simulink model "VehCtrlMdel241025_2018b_amkspdlimit"  (R2019b)
settings: Solver=FixedStepDiscrete  StartTime=0.0  StopTime=30  FixedStep=0.0005  RelTol=1e-3  EnableMultiTasking=on
values from neighbouring files (symbols this model uses):
  Ldwf = 0.4    [VxSpdEstiPara.m]
  Ldwr = 0.5    [VxSpdEstiPara.m]
  thr1 = 0.5    [VxSpdEstiPara.m]
  thr2 = 0.5    [VxSpdEstiPara.m]
  thr3 = 0.5    [VxSpdEstiPara.m]
  thr4 = 0.5    [VxSpdEstiPara.m]
  TrqRquRate = 20    [VxSpdEstiPara.m]
undefined symbols (not defined in the file or in its folder): Ax_OffSet, Ay_OffSet, Caf, Car, DiscIntNeverNeededParam, dwf, dwr, h, i1, i2, I_AN06_5V, I_AN07_5V, I_AN08_5V, I_AN09_5V, I_AN10_5V, I_SW01_L, I_SW02_L, I_SW03_L, I_SW05_L, I_SW07_L, Iz, Kc, Ki, Kp, lf, lr, m, O_SW01_LS0A4, O_SW02_LS0A4, O_SW04_LS0A4, O_SW05_LS0A4, O_SW06_LS0A4, O_SW07_LS0A4, O_SW08_LS0A4, O_SW09_LS0A4, O_SW12_HS1A, O_SW13_HS1A, O_SW14_HS1A, O_SW15_HS1A, Offset_Angle, PWM3, Qa, Ra, RearRatio, Rt, thr5, YawRate_OffSet
libraries: simulink x159, ec5744lib x142, canmsglib x18, MyDesignedModel x1
(part 5 of 6)

== system VehCtrlMdel241025_2018b_amkspdlimit/Input/EMRAXMCU_RECIEVE/MCU_pwr/MCU_VCUMeter1 ==
  ID : Inport
  Msg : Inport  Port=2
  Enable : EnablePort
  CAN Unpack : canmsglib/CAN Unpack  CANdbFile=E:\candbc\MCU_No1.dbc  MsgList=(none)  MsgName=MCU2VCU2_ID1  MsgIDType=Extended (29-bit identifier)  MsgIdentifier=218089455  MsgLength=8  SignalInfo={'MCU2VCU2_Current_AC_Feedback_ID1','48','16','LE','unsigned','Standard','0','1.000000e-01','-1600','-1600','1600';'MCU2VCU2_Current_DC_feedback_ID1','32','16','LE','unsigned','Standard','0','1.000000e-01','-1600','-1600','1600';'MCU2VCU2_MCU_Temp_ID1','0','8','LE','unsigned','Standard','0','1','-50','-50','200';'MCU2VCU2_Motor_Temp_ID1','8','8','LE','unsigned','Standard','0','1','-50','-50','200';'MCU2VCU2_Voltage_Feedback_ID1','16','16','LE','unsigned','Standard','0','1.000000e-01','0','0','1000'}  IDPort=off  TimestampPort=off  ErrorPort=off  RemotePort=off  LengthPort=off  StatusPort=off  ApplyMinMax=off
      settings: SourceProductName=Vehicle Network Toolbox  SourceProductBaseCode=VN  DataFormat=CANdb specified signals
  CANUnPackMessage4 : ec5744lib/RapidECU_U3/04CANCommunication/CANUnPackMessage  datalength=8  canmessagetype=Extended(29-bit ID)  sampletime=-1
      settings: SourceProductName=ECUCoder for MPC5744
  MeaModule1 : ec5744lib/RapidECU_U3/07Calibration/MeaModule  signal=AC_current
      settings: SourceProductName=ECUCoder for MPC5744
  MeaModule2 : ec5744lib/RapidECU_U3/07Calibration/MeaModule  signal=DC_current
      settings: SourceProductName=ECUCoder for MPC5744
  MeaModule3 : ec5744lib/RapidECU_U3/07Calibration/MeaModule  signal=MCU_Temp
      settings: SourceProductName=ECUCoder for MPC5744
  MeaModule4 : ec5744lib/RapidECU_U3/07Calibration/MeaModule  signal=motor_Temp
      settings: SourceProductName=ECUCoder for MPC5744
  MeaModule5 : ec5744lib/RapidECU_U3/07Calibration/MeaModule  signal=voltage
      settings: SourceProductName=ECUCoder for MPC5744
  "AC_current " : Outport
  MCU_temp : Outport  Port=2
  current : Outport  Port=3
  motor_temp : Outport  Port=4
  voltage : Outport  Port=5
  wires:
  Msg/1 -> CANUnPackMessage4/2
  ID/1 -> CANUnPackMessage4/1
  CANUnPackMessage4/1 -> CAN Unpack/1
  CAN Unpack/1 -> MeaModule1/1  "AC_current"
  CAN Unpack/5 -> MeaModule5/1  "voltage"
  CAN Unpack/4 -> MeaModule4/1  "moter_temp"
  MeaModule1/1 -> "AC_current "/1
  MeaModule2/1 -> current/1
  CAN Unpack/3 -> MeaModule3/1  "MCU_temp"
  CAN Unpack/2 -> MeaModule2/1  "DC_current"
  MeaModule3/1 -> MCU_temp/1
  MeaModule4/1 -> motor_temp/1
  MeaModule5/1 -> voltage/1

== system VehCtrlMdel241025_2018b_amkspdlimit/Input/EMRAXMCU_RECIEVE/MCU_state/MCU_state ==
  ID : Inport
  Msg : Inport  Port=2
  Enable : EnablePort
  CAN Unpack : canmsglib/CAN Unpack  CANdbFile=E:\candbc\MCU_No1.dbc  MsgList=(none)  MsgName=MCU2VCU1_ID1  MsgIDType=Extended (29-bit identifier)  MsgIdentifier=218089199  MsgLength=8  SignalInfo={'MCU2VCU1_12V_error_ID1','45','1','LE','unsigned','Standard','0','1','0','0','1';'MCU2VCU1_Error_All_ID1','56','2','LE','unsigned','Standard','0','1','0','0','3';'MCU2VCU1_LowVoltage_error_ID1','46','1','LE','unsigned','Standard','0','1','0','0','1';'MCU2VCU1_MCU_Ready_ID1','40','1','LE','unsigned','Standard','0','1','0','0','1';'MCU2VCU1_MCU_Temp_error_ID1','48','1','LE','unsigned','Standard','0','1','0','0','1';'MCU2VCU1_Mode_Feedback_ID1','32','8','LE','unsigned','Standard','0','1','0','0','255';'MCU2VCU1_MotorTemp_error_ID1','49','1','LE','unsigned','Standard','0','1','0','0','1';'MCU2VCU1_OverCurrent_error_ID1','43','1','LE','unsigned','Standard','0','1','0','0','1';'MCU2VCU1_OverPower_error_ID1','47','1','LE','unsigned','Standard','0','1','0','0','1';'MCU2VCU1_OverVoltage_error_ID1','44','1','LE','unsigned','Standard','0','1','0','0','1';'MCU2VCU1_PrechargeState_ID1','41','1','LE','unsigned','Standard','0','1','0','0','1';'MCU2VCU1_Reslove_Error_ID1','42','1','LE','unsigned','Standard','0','1','0','0','1';'MCU2VCU1_Selfcheck_ID1','55','1','LE','unsigned','Standard','0','1','0','0','1';'MCU2VCU1_Speed_Feedback_ID1','0','16','LE','unsigned','Standard','0','5.000000e-01','-10000','-10000','10000';'MCU2VCU1_Torque_Feedback_ID1','16','16','LE','unsigned','Standard','0','1','0','0','1000'}  IDPort=off  TimestampPort=off  ErrorPort=off  RemotePort=off  LengthPort=off  StatusPort=off  ApplyMinMax=off
      settings: SourceProductName=Vehicle Network Toolbox  SourceProductBaseCode=VN  DataFormat=CANdb specified signals
  CANUnPackMessage4 : ec5744lib/RapidECU_U3/04CANCommunication/CANUnPackMessage  datalength=8  canmessagetype=Extended(29-bit ID)  sampletime=-1
      settings: SourceProductName=ECUCoder for MPC5744
  MeaModule : ec5744lib/RapidECU_U3/07Calibration/MeaModule  signal=RPM
      settings: SourceProductName=ECUCoder for MPC5744
  MeaModule1 : ec5744lib/RapidECU_U3/07Calibration/MeaModule  signal=alarm
      settings: SourceProductName=ECUCoder for MPC5744
  MeaModule2 : ec5744lib/RapidECU_U3/07Calibration/MeaModule  signal=L12V_error
      settings: SourceProductName=ECUCoder for MPC5744
  MeaModule3 : ec5744lib/RapidECU_U3/07Calibration/MeaModule  signal=controller_ready
      settings: SourceProductName=ECUCoder for MPC5744
  MeaModule5 : ec5744lib/RapidECU_U3/07Calibration/MeaModule  signal=selfcheck
      settings: SourceProductName=ECUCoder for MPC5744
  MeaModule6 : ec5744lib/RapidECU_U3/07Calibration/MeaModule  signal=trq
      settings: SourceProductName=ECUCoder for MPC5744
  12V_error : Outport
  alarm : Outport  Port=2
  undervol : Outport  Port=3
  controller_ready : Outport  Port=4
  MCU_temp_warn : Outport  Port=5
  mode_cmd8 : Outport  Port=6
  motor_temp_warn : Outport  Port=7
  overcur : Outport  Port=8
  pow_lim_warn : Outport  Port=9
  overvol : Outport  Port=10
  precharge : Outport  Port=11
  rotation_warn : Outport  Port=12
  selfcech : Outport  Port=13
  RPM : Outport  Port=14
  torque : Outport  Port=15
  wires:
  Msg/1 -> CANUnPackMessage4/2
  ID/1 -> CANUnPackMessage4/1
  CANUnPackMessage4/1 -> CAN Unpack/1
  MeaModule/1 -> RPM/1  "RPM"
  MeaModule1/1 -> alarm/1
  MeaModule2/1 -> 12V_error/1
  MeaModule3/1 -> controller_ready/1
  MeaModule5/1 -> selfcech/1
  MeaModule6/1 -> torque/1  "Trq"
  CAN Unpack/14 -> MeaModule/1  "RPM"
  CAN Unpack/15 -> MeaModule6/1  "Trq"
  CAN Unpack/13 -> MeaModule5/1
  CAN Unpack/11 -> precharge/1  "Precharge"
  CAN Unpack/10 -> overvol/1  "overvol"
  CAN Unpack/9 -> pow_lim_warn/1  "overpower"
  CAN Unpack/8 -> overcur/1  "overCurrent"
  CAN Unpack/7 -> motor_temp_warn/1  "motorTemp_error"
  CAN Unpack/6 -> mode_cmd8/1  "Mode"
  CAN Unpack/5 -> MCU_temp_warn/1  "MCU_Temp_error"
  CAN Unpack/4 -> MeaModule3/1  "MCU_Ready"
  CAN Unpack/3 -> undervol/1  "low_VOL"
  CAN Unpack/2 -> MeaModule1/1  "Error_ALL"
  CAN Unpack/1 -> MeaModule2/1  "12V_error"
  CAN Unpack/12 -> rotation_warn/1  "Reslove_error"

== system VehCtrlMdel241025_2018b_amkspdlimit/Input/IMU_Recieve/IMU_state/MCU_state ==
  ID : Inport
  Msg : Inport  Port=2
  Enable : EnablePort
  CAN Unpack : canmsglib/CAN Unpack  CANdbFile=d:\Users\YJR\Desktop\IMU.dbc  MsgList=(none)  MsgName=IMU  MsgIDType=Standard (11-bit identifier)  MsgIdentifier=513  MsgLength=8  SignalInfo={'IMU_Ax_Valid','1','1','LE','unsigned','Standard','0','1','0','-Inf','Inf';'IMU_Ax_Value','40','16','LE','unsigned','Standard','0','1.500000e-04','-4.915200e+00','-Inf','Inf';'IMU_Ay_Valid','2','1','LE','unsigned','Standard','0','1','0','-Inf','Inf';'IMU_Ay_Value','24','16','LE','unsigned','Standard','0','1.500000e-04','-4.915200e+00','-Inf','Inf';'IMU_DTC','4','4','LE','unsigned','Standard','0','1','0','-Inf','Inf';'IMU_Yaw_Valid','3','1','LE','unsigned','Standard','0','1','0','-Inf','Inf';'IMU_Yaw_Value','8','16','LE','unsigned','Standard','0','5.710000e-03','-1.872400e+02','-Inf','Inf'}  IDPort=off  TimestampPort=off  ErrorPort=off  RemotePort=off  LengthPort=off  StatusPort=off  ApplyMinMax=off
      settings: SourceProductName=Simulink Real-Time  SourceProductBaseCode=XP  DataFormat=CANdb specified signals
  CANUnPackMessage4 : ec5744lib/RapidECU_U3/04CANCommunication/CANUnPackMessage  datalength=8  canmessagetype=Standard(11-bit ID)  sampletime=-1
      settings: SourceProductName=ECUCoder for MPC5744
  MeaModule2 : ec5744lib/RapidECU_U3/07Calibration/MeaModule  signal=IMU_Ay_Value
      settings: SourceProductName=ECUCoder for MPC5744
  MeaModule3 : ec5744lib/RapidECU_U3/07Calibration/MeaModule  signal=IMU_Yaw_Value
      settings: SourceProductName=ECUCoder for MPC5744
  MeaModule4 : ec5744lib/RapidECU_U3/07Calibration/MeaModule  signal=IMU_Ax_Value
      settings: SourceProductName=ECUCoder for MPC5744
  IMU_Ax_Value : Outport  VectorParamsAs1DForOutWhenUnconnected=off
  IMU_Ay_Value : Outport  Port=2  VectorParamsAs1DForOutWhenUnconnected=off
  IMU_Yaw_Value : Outport  Port=3  VectorParamsAs1DForOutWhenUnconnected=off
  IMU_Ay_Valid : Outport  Port=4  VectorParamsAs1DForOutWhenUnconnected=off
  IMU_DTC : Outport  Port=5  VectorParamsAs1DForOutWhenUnconnected=off
  IMU_Yaw_Valid : Outport  Port=6  VectorParamsAs1DForOutWhenUnconnected=off
  IMU_Ax_Valid : Outport  Port=7  VectorParamsAs1DForOutWhenUnconnected=off
  wires:
  Msg/1 -> CANUnPackMessage4/2
  ID/1 -> CANUnPackMessage4/1
  CANUnPackMessage4/1 -> CAN Unpack/1
  CAN Unpack/2 -> MeaModule2/1
  CAN Unpack/3 -> IMU_Ay_Valid/1
  CAN Unpack/4 -> MeaModule4/1
  CAN Unpack/5 -> IMU_DTC/1
  CAN Unpack/7 -> MeaModule3/1
  CAN Unpack/6 -> IMU_Yaw_Valid/1
  CAN Unpack/1 -> IMU_Ax_Valid/1
  MeaModule2/1 -> IMU_Ax_Value/1
  MeaModule3/1 -> IMU_Yaw_Value/1
  MeaModule4/1 -> IMU_Ay_Value/1

== system VehCtrlMdel241025_2018b_amkspdlimit/Input/StrSnis_Receive/StrWhSnis_state/IMU_state ==
  ID : Inport
  Msg : Inport  Port=2
  Enable : EnablePort
  CAN Unpack : canmsglib/CAN Unpack  Commented=on  CANdbFile=d:\Users\YJR\Desktop\DBC\SWAS_3.dbc  MsgList=(none)  MsgName=PPEI_Steering_Wheel_Angle  MsgIDType=Standard (11-bit identifier)  MsgIdentifier=330  MsgLength=8  SignalInfo={'SAS_CheckSum','36','4','LE','unsigned','Standard','0','1','0','-Inf','Inf';'SAS_MassageCounter','32','4','LE','unsigned','Standard','0','1','0','0','15';'SAS_TrimmingFlag','26','1','LE','unsigned','Standard','0','1','0','0','255';'StrWhAng','8','16','BE','unsigned','Standard','0','1','0','0','65535';'StrWhAngV','16','8','LE','unsigned','Standard','0','1','0','0','1';'StrWhlAngSenCalFlag','25','1','LE','unsigned','Standard','0','1','0','0','3';'StrngWhlAngSnsrFailFlag','24','1','LE','unsigned','Standard','0','1','0','0','1'}  IDPort=off  TimestampPort=off  ErrorPort=off  RemotePort=off  LengthPort=off  StatusPort=off  ApplyMinMax=off
      settings: SourceProductName=Simulink Real-Time  SourceProductBaseCode=XP  DataFormat=CANdb specified signals
  CAN Unpack1 : canmsglib/CAN Unpack  CANdbFile=d:\Users\YJR\Desktop\DBC\SWAS.dbc  MsgList=(none)  MsgName=PPEI_Steering_Wheel_Angle  MsgIDType=Standard (11-bit identifier)  MsgIdentifier=330  MsgLength=8  SignalInfo={'StWhlAngAliveRollCnt','0','8','BE','unsigned','Standard','0','1','0','0','63';'StrWhAng','32','16','BE','unsigned','Standard','0','0.1','-779.3','-779.3','5774.2';'StrWhAngV','16','8','BE','unsigned','Standard','0','1','0','0','255'}  IDPort=off  TimestampPort=off  ErrorPort=off  RemotePort=off  LengthPort=off  StatusPort=off  ApplyMinMax=off
      settings: SourceProductName=Simulink Real-Time  SourceProductBaseCode=XP  DataFormat=CANdb specified signals
  CANUnPackMessage4 : ec5744lib/RapidECU_U3/04CANCommunication/CANUnPackMessage  datalength=8  canmessagetype=Standard(11-bit ID)  sampletime=-1
      settings: SourceProductName=ECUCoder for MPC5744
  MeaModule1 : ec5744lib/RapidECU_U3/07Calibration/MeaModule  signal=StrWhlAngAliveRollCnt
      settings: SourceProductName=ECUCoder for MPC5744
  MeaModule2 : ec5744lib/RapidECU_U3/07Calibration/MeaModule  signal=StrWhlAng
      settings: SourceProductName=ECUCoder for MPC5744
  MeaModule3 : ec5744lib/RapidECU_U3/07Calibration/MeaModule  signal=StrWhlAngV
      settings: SourceProductName=ECUCoder for MPC5744
  StrWhlAng : Outport  VectorParamsAs1DForOutWhenUnconnected=off
  StrWhlAngV : Outport  Port=2  VectorParamsAs1DForOutWhenUnconnected=off
  StrWhlAngAliveRollCnt : Outport  Port=3  VectorParamsAs1DForOutWhenUnconnected=off
  wires:
  Msg/1 -> CANUnPackMessage4/2
  ID/1 -> CANUnPackMessage4/1
  CANUnPackMessage4/1 -> CAN Unpack1/1
  CAN Unpack1/1 -> MeaModule1/1
  CAN Unpack1/2 -> MeaModule2/1
  CAN Unpack1/3 -> MeaModule3/1
  MeaModule1/1 -> StrWhlAngAliveRollCnt/1
  MeaModule2/1 -> StrWhlAng/1
  MeaModule3/1 -> StrWhlAngV/1

== system VehCtrlMdel241025_2018b_amkspdlimit/Input_Processing/Function-Call Subsystem/IMU/Subsystem ==
  note: 定义数据类型
  IMU_Ax_Value : Inport
  IMU_Ay_Value : Inport  Port=2
  IMU_Yaw_Value : Inport  Port=3
  Add{,1..5} (6 alike) : Sum
  Constant : Constant  Value=5000
  Constant1 : Constant  Value=-5000
  Constant10 : Constant  Value=200  SampleTime=-1
  Constant11 : Constant  Value=-200  SampleTime=-1
  Constant12 : Constant  Value=Ax_OffSet
  Constant13 : Constant  Value=Ay_OffSet
  Constant14 : Constant  Value=YawRate_OffSet
  Constant15 : Constant  Value=Offset_Angle
  Constant16 : Constant  Value=Offset_Angle
  Constant2 : Constant  Value=5000
  Constant3 : Constant  Value=5000
  Constant4 : Constant  Value=-5000
  Constant5 : Constant  Value=-5000
  Constant6 : Constant  Value=1.5  SampleTime=-1
  Constant7 : Constant  Value=-1.5  SampleTime=-1
  Constant8 : Constant  Value=1.5  SampleTime=-1
  Constant9 : Constant  Value=-1.5  SampleTime=-1
  Cos : Trigonometry  Operator=cos
  Cos1 : Trigonometry  Operator=cos
  Gain : Gain  Gain=0.7
  Gain1 : Gain  Gain=0.3
  Gain2 : Gain  Gain=0.7
  Gain3 : Gain  Gain=0.3
  Gain4 : Gain  Gain=0.7
  Gain5 : Gain  Gain=0.3
  Product : Product
  Product1 : Product
  Rate Limiter Dynamic : simulink/Discontinuities/Rate Limiter Dynamic
      settings: SourceProductName=Simulink
  Rate Limiter Dynamic1 : simulink/Discontinuities/Rate Limiter Dynamic
      settings: SourceProductName=Simulink
  Rate Limiter Dynamic2 : simulink/Discontinuities/Rate Limiter Dynamic
      settings: SourceProductName=Simulink
  Saturation Dynamic : simulink/Discontinuities/Saturation Dynamic  OutMin=[]  OutMax=[]  OutDataTypeStr=Inherit: Same as second input  OutDataType=fixdt(1, 16)  OutScaling=2^-10  DoSatur=off
  Saturation Dynamic1 : simulink/Discontinuities/Saturation Dynamic  OutMin=[]  OutMax=[]  OutDataTypeStr=Inherit: Same as second input  OutDataType=fixdt(1, 16)  OutScaling=2^-10  DoSatur=off
  Saturation Dynamic2 : simulink/Discontinuities/Saturation Dynamic  OutMin=[]  OutMax=[]  OutDataTypeStr=Inherit: Same as second input  OutDataType=fixdt(1, 16)  OutScaling=2^-10  DoSatur=off
  Saturation2 : Saturate  UpperLimit=180  LowerLimit=-180
  Unit Delay : UnitDelay  SampleTime=-1  HasFrameUpgradeWarning=on
  Unit Delay1 : UnitDelay  SampleTime=-1  HasFrameUpgradeWarning=on
  Unit Delay2 : UnitDelay  SampleTime=-1  HasFrameUpgradeWarning=on
  IMU_Ax_Value_out : Outport  VectorParamsAs1DForOutWhenUnconnected=off
  IMU_Ay_Value_out : Outport  Port=2  VectorParamsAs1DForOutWhenUnconnected=off
  IMU_Yaw_Value_out : Outport  Port=3  VectorParamsAs1DForOutWhenUnconnected=off
  wires:
  IMU_Ay_Value/1 -> Unit Delay1/1, Gain2/1  "Ay"
  Unit Delay/1 -> Gain1/1
  Gain/1 -> Add2/2
  Constant2/1 -> Rate Limiter Dynamic1/1
  Constant/1 -> Rate Limiter Dynamic/1
  Add2/1 -> Rate Limiter Dynamic/2
  Gain2/1 -> Add1/1
  IMU_Yaw_Value/1 -> Gain4/1, Unit Delay2/1  "YawRate"
  Gain1/1 -> Add2/1
  Gain5/1 -> Add3/2
  IMU_Ax_Value/1 -> Gain/1, Unit Delay/1  "Ax"
  Constant11/1 -> Saturation Dynamic2/3
  Add1/1 -> Rate Limiter Dynamic1/2
  Unit Delay1/1 -> Gain3/1
  Constant8/1 -> Saturation Dynamic1/1
  Add3/1 -> Rate Limiter Dynamic2/2
  Constant4/1 -> Rate Limiter Dynamic1/3
  Rate Limiter Dynamic1/1 -> Saturation Dynamic1/2
  Constant1/1 -> Rate Limiter Dynamic/3
  Gain4/1 -> Add3/1
  Constant7/1 -> Saturation Dynamic/3
  Constant3/1 -> Rate Limiter Dynamic2/1
  Product/1 -> IMU_Ax_Value_out/1  "IMU_Ax_Value"
  Constant9/1 -> Saturation Dynamic1/3
  Add5/1 -> IMU_Yaw_Value_out/1  "IMU_Yaw_Value"
  Rate Limiter Dynamic2/1 -> Saturation2/1
  Saturation2/1 -> Saturation Dynamic2/2  "IMU_Yaw_Value"
  Constant10/1 -> Saturation Dynamic2/1
  Constant5/1 -> Rate Limiter Dynamic2/3
  Rate Limiter Dynamic/1 -> Saturation Dynamic/2
  Gain3/1 -> Add1/2
  Product1/1 -> IMU_Ay_Value_out/1  "IMU_Ay_Value"
  Constant6/1 -> Saturation Dynamic/1
  Unit Delay2/1 -> Gain5/1
  Saturation Dynamic/1 -> Add/1  "IMU_Ax_Value"
  Constant12/1 -> Add/2
  Saturation Dynamic1/1 -> Add4/1  "IMU_Ay_Value"
  Constant13/1 -> Add4/2
  Saturation Dynamic2/1 -> Add5/1  "IMU_Yaw_Value"
  Constant14/1 -> Add5/2
  Add/1 -> Product/1
  Cos/1 -> Product/2
  Constant15/1 -> Cos/1
  Constant16/1 -> Cos1/1
  Cos1/1 -> Product1/2
  Add4/1 -> Product1/1

== system VehCtrlMdel241025_2018b_amkspdlimit/Input_Processing/Subsystem/WhlSlpageJudgment/加速度差判断 ==
  note: 输出“1”代表判定有效
  <VxFL_mps> : Inport
  <VxFR_mps> : Inport  Port=2
  <VxRL_mps> : Inport  Port=3
  <VxRR_mps> : Inport  Port=4
  IMU_Ax_mpss : Inport  Port=5
  Abs{,1..3} (4 alike) : Abs
  Add{,1..3} (4 alike) : Sum  Inputs=+-
  Add{4..7} (4 alike) : Sum  Inputs=-+
  Compare To Constant{,1..3} (4 alike) : simulink/Logic and Bit Operations/Compare To Constant  relop=<=  const=thr2  OutDataTypeStr=boolean
  Divide{,1..3} (4 alike) : Product  Inputs=*/
  Filter : Subsystem
  Filter1 : Subsystem
  Filter2 : Subsystem
  Filter3 : Subsystem
  Unit Delay{,1..3} (4 alike) : UnitDelay  SampleTime=-1  HasFrameUpgradeWarning=on
  steptime{,1..3} (4 alike) : Constant  Value=single(0.01)
  y : Outport
  y1 : Outport  Port=2
  y2 : Outport  Port=3
  y3 : Outport  Port=4
  wires:
  Compare To Constant/1 -> y/1
  Compare To Constant2/1 -> y2/1
  Abs2/1 -> Compare To Constant2/1
  Add1/1 -> Abs1/1
  Abs/1 -> Compare To Constant/1
  [IMU_Ax_mpss] -> Add3/2
  [IMU_Ax_mpss] -> Add2/2
  [IMU_Ax_mpss] -> Add/2
  Abs3/1 -> Compare To Constant3/1
  Compare To Constant3/1 -> y3/1
  Compare To Constant1/1 -> y1/1
  [IMU_Ax_mpss] -> Add1/2
  Add/1 -> Abs/1
  Add3/1 -> Abs3/1
  Abs1/1 -> Compare To Constant1/1
  Add2/1 -> Abs2/1
  <VxFL_mps>/1 -> Add4/2, Unit Delay/1
  Unit Delay/1 -> Add4/1
  Add4/1 -> Divide/1
  steptime/1 -> Divide/2
  Divide/1 -> Filter/1(In)
  IMU_Ax_mpss/1 -> [IMU_Ax_mpss]
  steptime1/1 -> Divide1/2
  Add5/1 -> Divide1/1
  Unit Delay1/1 -> Add5/1
  <VxFR_mps>/1 -> Unit Delay1/1, Add5/2
  Divide1/1 -> Filter1/1(In)
  steptime2/1 -> Divide2/2
  Add6/1 -> Divide2/1
  Unit Delay2/1 -> Add6/1
  <VxRL_mps>/1 -> Unit Delay2/1, Add6/2
  Divide2/1 -> Filter2/1(In)
  steptime3/1 -> Divide3/2
  Add7/1 -> Divide3/1
  Unit Delay3/1 -> Add7/1
  <VxRR_mps>/1 -> Unit Delay3/1, Add7/2
  Divide3/1 -> Filter3/1(In)
  Filter/1(Out) -> Add/1
  Filter1/1(Out) -> Add1/1
  Filter2/1(Out) -> Add2/1
  Filter3/1(Out) -> Add3/1

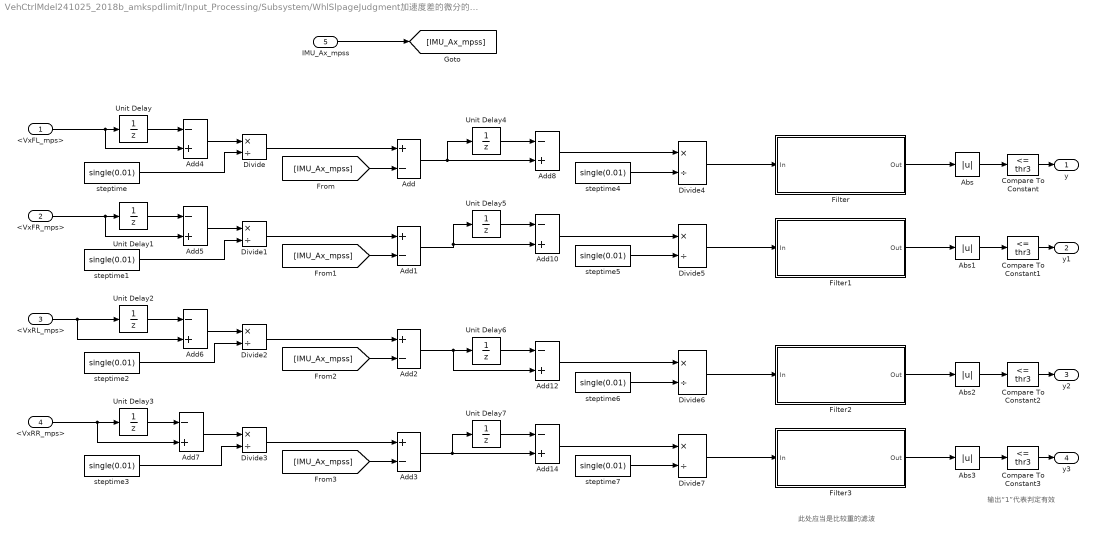
== system VehCtrlMdel241025_2018b_amkspdlimit/Input_Processing/Subsystem/WhlSlpageJudgment/加速度差的微分的判断 ==
  note: 此处应当是比较重的滤波
  note: 输出“1”代表判定有效
  <VxFL_mps> : Inport
  <VxFR_mps> : Inport  Port=2
  <VxRL_mps> : Inport  Port=3
  <VxRR_mps> : Inport  Port=4
  IMU_Ax_mpss : Inport  Port=5
  Abs{,1..3} (4 alike) : Abs
  Add{,1..3} (4 alike) : Sum  Inputs=+-
  Add{4..8,10,12,14} (8 alike) : Sum  Inputs=-+
  Compare To Constant{,1..3} (4 alike) : simulink/Logic and Bit Operations/Compare To Constant  relop=<=  const=thr3  OutDataTypeStr=boolean
  Divide{,1..7} (8 alike) : Product  Inputs=*/
  Filter : Subsystem
  Filter1 : Subsystem
  Filter2 : Subsystem
  Filter3 : Subsystem
  Unit Delay{,1..7} (8 alike) : UnitDelay  SampleTime=-1  HasFrameUpgradeWarning=on
  steptime{,1..7} (8 alike) : Constant  Value=single(0.01)
  y : Outport
  y1 : Outport  Port=2
  y2 : Outport  Port=3
  y3 : Outport  Port=4
  wires:
  Divide3/1 -> Add3/1
  <VxRR_mps>/1 -> Add7/2, Unit Delay3/1
  Unit Delay3/1 -> Add7/1
  Add7/1 -> Divide3/1
  steptime3/1 -> Divide3/2
  Divide2/1 -> Add2/1
  <VxRL_mps>/1 -> Add6/2, Unit Delay2/1
  Unit Delay2/1 -> Add6/1
  Add6/1 -> Divide2/1
  steptime2/1 -> Divide2/2
  Divide1/1 -> Add1/1
  <VxFR_mps>/1 -> Add5/2, Unit Delay1/1
  Unit Delay1/1 -> Add5/1
  Add5/1 -> Divide1/1
  steptime1/1 -> Divide1/2
  IMU_Ax_mpss/1 -> [IMU_Ax_mpss]
  Divide/1 -> Add/1
  steptime/1 -> Divide/2
  Add4/1 -> Divide/1
  Unit Delay/1 -> Add4/1
  <VxFL_mps>/1 -> Unit Delay/1, Add4/2
  Abs1/1 -> Compare To Constant1/1
  [IMU_Ax_mpss] -> Add1/2
  Compare To Constant1/1 -> y1/1
  Compare To Constant3/1 -> y3/1
  Abs3/1 -> Compare To Constant3/1
  [IMU_Ax_mpss] -> Add/2
  [IMU_Ax_mpss] -> Add2/2
  [IMU_Ax_mpss] -> Add3/2
  Abs/1 -> Compare To Constant/1
  Abs2/1 -> Compare To Constant2/1
  Compare To Constant2/1 -> y2/1
  Compare To Constant/1 -> y/1
  Add/1 -> Add8/2, Unit Delay4/1
  Unit Delay4/1 -> Add8/1
  Add8/1 -> Divide4/1
  steptime4/1 -> Divide4/2
  Divide4/1 -> Filter/1(In)
  steptime5/1 -> Divide5/2
  Add10/1 -> Divide5/1
  Unit Delay5/1 -> Add10/1
  Add1/1 -> Unit Delay5/1, Add10/2
  Divide5/1 -> Filter1/1(In)
  Divide6/1 -> Filter2/1(In)
  Add2/1 -> Add12/2, Unit Delay6/1
  Add12/1 -> Divide6/1
  steptime6/1 -> Divide6/2
  Unit Delay6/1 -> Add12/1
  steptime7/1 -> Divide7/2
  Add14/1 -> Divide7/1
  Add3/1 -> Unit Delay7/1, Add14/2
  Unit Delay7/1 -> Add14/1
  Divide7/1 -> Filter3/1(In)
  Filter/1(Out) -> Abs/1
  Filter1/1(Out) -> Abs1/1
  Filter2/1(Out) -> Abs2/1
  Filter3/1(Out) -> Abs3/1

== system VehCtrlMdel241025_2018b_amkspdlimit/Input_Processing/Subsystem/WhlSlpageJudgment/速差判断 ==
  note: 输出“1”代表判定有效
  <VxFL_mps> : Inport
  <VxFR_mps> : Inport  Port=2
  <VxRL_mps> : Inport  Port=3
  <VxRR_mps> : Inport  Port=4
  VehSpd_mps : Inport  Port=5
  In6 : Inport  Port=6
  AND{,1..3} (4 alike) : Logic  AllPortsSameDT=off  OutDataTypeStr=boolean
  Abs{,1..3} (4 alike) : Abs
  Add{,1..3} (4 alike) : Sum  Inputs=+-
  Bus Selector1 : BusSelector  OutputSignals=WhlSpdii_mps.WhlSpdRL_Valid,WhlSpdii_mps.WhlSpdRR_Valid,WhlSpdii_mps.WhlSpdFR_Valid,WhlSpdii_mps.WhlSpdFL_Valid
  Compare To Constant{,1..3} (4 alike) : simulink/Logic and Bit Operations/Compare To Constant  relop=<=  const=thr1  OutDataTypeStr=boolean
  y : Outport
  y1 : Outport  Port=2
  y2 : Outport  Port=3
  y3 : Outport  Port=4
  wires:
  Add2/1 -> Abs2/1
  Abs1/1 -> Compare To Constant1/1
  <VxRR_mps>/1 -> Add3/1
  Add3/1 -> Abs3/1
  Add/1 -> Abs/1
  [VehSpd_mps] -> Add1/2
  <VxRL_mps>/1 -> Add2/1
  <VxFR_mps>/1 -> Add1/1
  Compare To Constant1/1 -> AND2/1
  Compare To Constant3/1 -> AND1/1
  Abs3/1 -> Compare To Constant3/1
  [VehSpd_mps] -> Add/2
  [VehSpd_mps] -> Add2/2
  [VehSpd_mps] -> Add3/2
  Abs/1 -> Compare To Constant/1
  Add1/1 -> Abs1/1
  Abs2/1 -> Compare To Constant2/1
  <VxFL_mps>/1 -> Add/1
  Compare To Constant2/1 -> AND/1
  Compare To Constant/1 -> AND3/1
  VehSpd_mps/1 -> [VehSpd_mps]
  In6/1 -> Bus Selector1/1
  Bus Selector1/1 -> AND/2  "<WhlSpdRL_Valid>"
  Bus Selector1/2 -> AND1/2  "<WhlSpdRR_Valid>"
  Bus Selector1/3 -> AND2/2  "<WhlSpdFR_Valid>"
  Bus Selector1/4 -> AND3/2  "<WhlSpdFL_Valid>"
  AND3/1 -> y/1
  AND2/1 -> y1/1
  AND1/1 -> y3/1
  AND/1 -> y2/1

== system VehCtrlMdel241025_2018b_amkspdlimit/Input_Processing/Subsystem/WhlSpdSelect/Filter ==
  In : Inport
  Add : Sum
  Constant : Constant  Value=single(0)
  Constant1 : Constant  Value=single(100)
  Constant2 : Constant  Value=single(15)
  Constant3 : Constant  Value=single(-15)
  Gain : Gain  Gain=0
  Gain1 : Gain
  Rate Limiter Dynamic : simulink/Discontinuities/Rate Limiter Dynamic
      settings: SourceProductName=Simulink
  Saturation Dynamic : simulink/Discontinuities/Saturation Dynamic  OutMin=[]  OutMax=[]  OutDataTypeStr=Inherit: Same as second input  OutDataType=fixdt(1, 16)  OutScaling=2^-10  DoSatur=off
  Unit Delay : UnitDelay  SampleTime=-1  HasFrameUpgradeWarning=on
  VehVxEst_mps : Outport
  wires:
  In/1 -> Saturation Dynamic/2
  Saturation Dynamic/1 -> Rate Limiter Dynamic/2
  Constant1/1 -> Saturation Dynamic/1
  Constant/1 -> Saturation Dynamic/3
  Unit Delay/1 -> Gain/1
  Gain/1 -> Add/1
  Gain1/1 -> Add/2
  Rate Limiter Dynamic/1 -> Gain1/1, Unit Delay/1
  Add/1 -> VehVxEst_mps/1
  Constant2/1 -> Rate Limiter Dynamic/1
  Constant3/1 -> Rate Limiter Dynamic/3

== system VehCtrlMdel241025_2018b_amkspdlimit/Input_Processing/Subsystem/WhlSpdSelect/Subsystem ==
  <VxFL_mps> : Inport
  <VxFR_mps> : Inport  Port=2
  <VxRL_mps> : Inport  Port=3
  <VxRR_mps> : Inport  Port=4
  Add3 : Sum  Inputs=++++
  Add4 : Sum  Inputs=+--
  Gain1 : Gain  Gain=1/2
  Min3 : MinMax  Function=max  Inputs=4
  Min4 : MinMax  Inputs=4
  Subsystem : Subsystem  Commented=on
  MiddleWhlSpd_mps : Outport
  wires:
  Add4/1 -> Gain1/1
  Add3/1 -> Add4/1
  Min3/1 -> Add4/3
  <VxRR_mps>/1 -> Min3/4, Add3/1, Min4/4
  <VxRL_mps>/1 -> Min3/3, Min4/3, Add3/2
  <VxFR_mps>/1 -> Min4/2, Min3/2, Add3/3
  Min4/1 -> Add4/2
  <VxFL_mps>/1 -> Add3/4, Min4/1, Min3/1
  Gain1/1 -> MiddleWhlSpd_mps/1  "MaxWhlSpd_mps"

== system VehCtrlMdel241025_2018b_amkspdlimit/Input/AMKMCU_Receive/FLAMKMCU/AMKMCU_state/MCU_state ==
  ID : Inport
  Msg : Inport  Port=2
  Enable : EnablePort
  Bus Creator : BusCreator  Inputs=12
  CAN Unpack : canmsglib/CAN Unpack  CANdbFile=d:\Users\YJR\Desktop\低压组\amk电机\DRe20_dbc_v1.16\DRe20_dbc_v1.16_CAN2.dbc  MsgList=(none)  MsgName=MCFL_ActualValue1  MsgIDType=Standard (11-bit identifier)  MsgIdentifier=640  MsgLength=8  SignalInfo={'MCFL_ActualTorque','32','16','LE','signed','Standard','0','0.0098','0','-Inf','Inf';'MCFL_ActualVelocity','48','16','LE','signed','Standard','0','1','0','-Inf','Inf';'MCFL_DCVoltage','16','16','LE','unsigned','Standard','0','1','0','-Inf','Inf';'MCFL_bDCOn','12','1','LE','unsigned','Standard','0','1','0','0','1';'MCFL_bDerating','15','1','LE','unsigned','Standard','0','1','0','0','1';'MCFL_bError','9','1','LE','unsigned','Standard','0','1','0','0','1';'MCFL_bInverterOn','14','1','LE','unsigned','Standard','0','1','0','0','1';'MCFL_bQuitDCOn','11','1','LE','unsigned','Standard','0','1','0','0','1';'MCFL_bQuitInverterOn','13','1','LE','unsigned','Standard','0','1','0','0','1';'MCFL_bReserve','0','8','LE','unsigned','Standard','0','1','0','0','255';'MCFL_bSystemReady','8','1','LE','unsigned','Standard','0','1','0','0','1';'MCFL_bWarn','10','1','LE','unsigned','Standard','0','1','0','0','1'}  IDPort=off  TimestampPort=off  ErrorPort=off  RemotePort=off  LengthPort=off  StatusPort=off  ApplyMinMax=off
      settings: SourceProductName=Simulink Real-Time  SourceProductBaseCode=XP  DataFormat=CANdb specified signals
  CANUnPackMessage4 : ec5744lib/RapidECU_U3/04CANCommunication/CANUnPackMessage  datalength=8  canmessagetype=Standard(11-bit ID)  sampletime=-1
      settings: SourceProductName=ECUCoder for MPC5744
  MeaModule1 : ec5744lib/RapidECU_U3/07Calibration/MeaModule  signal=MCFL_ActualVelocity
      settings: SourceProductName=ECUCoder for MPC5744
  MeaModule2 : ec5744lib/RapidECU_U3/07Calibration/MeaModule  signal=MCFL_DCVoltage
      settings: SourceProductName=ECUCoder for MPC5744
  MeaModule3 : ec5744lib/RapidECU_U3/07Calibration/MeaModule  signal=MCFL_bDCOn
      settings: SourceProductName=ECUCoder for MPC5744
  MeaModule4 : ec5744lib/RapidECU_U3/07Calibration/MeaModule  signal=MCFL_bError
      settings: SourceProductName=ECUCoder for MPC5744
  MeaModule5 : ec5744lib/RapidECU_U3/07Calibration/MeaModule  signal=MCFL_bInverterOn
      settings: SourceProductName=ECUCoder for MPC5744
  MeaModule6 : ec5744lib/RapidECU_U3/07Calibration/MeaModule  signal=MCFL_bQuitDCOn
      settings: SourceProductName=ECUCoder for MPC5744
  MeaModule7 : ec5744lib/RapidECU_U3/07Calibration/MeaModule  signal=MCFL_bQuitInverterOn
      settings: SourceProductName=ECUCoder for MPC5744
  MeaModule8 : ec5744lib/RapidECU_U3/07Calibration/MeaModule  signal=MCFL_bSystemReady
      settings: SourceProductName=ECUCoder for MPC5744
  MeaModule9 : ec5744lib/RapidECU_U3/07Calibration/MeaModule  signal=MCFL_ActualTorque
      settings: SourceProductName=ECUCoder for MPC5744
  FLAMKMCUtoVCU1 : Outport  VectorParamsAs1DForOutWhenUnconnected=off
  wires:
  Msg/1 -> CANUnPackMessage4/2
  ID/1 -> CANUnPackMessage4/1
  CANUnPackMessage4/1 -> CAN Unpack/1
  CAN Unpack/1 -> MeaModule9/1  "MCFL_ActualTorque"
  CAN Unpack/2 -> MeaModule1/1  "MCFL_ActualVelocity"
  CAN Unpack/3 -> MeaModule2/1  "MCFL_DCVoltage"
  CAN Unpack/4 -> MeaModule3/1  "MCFL_bDCOn"
  CAN Unpack/5 -> Bus Creator/5  "MCFL_bDerating"
  CAN Unpack/6 -> MeaModule4/1  "MCFL_bError"
  CAN Unpack/7 -> MeaModule5/1  "MCFL_bInverterOn"
  CAN Unpack/8 -> MeaModule6/1  "MCFL_bQuitDCOn"
  CAN Unpack/9 -> MeaModule7/1  "MCFL_bQuitInverterOn"
  CAN Unpack/10 -> Bus Creator/10  "MCFL_bReserve"
  CAN Unpack/11 -> MeaModule8/1  "MCFL_bSystemReady"
  CAN Unpack/12 -> Bus Creator/12  "MCFL_bWarn"
  Bus Creator/1 -> FLAMKMCUtoVCU1/1  "FLAMKMCUtoVCU1"
  MeaModule1/1 -> Bus Creator/2
  MeaModule2/1 -> Bus Creator/3
  MeaModule3/1 -> Bus Creator/4
  MeaModule4/1 -> Bus Creator/6
  MeaModule5/1 -> Bus Creator/7
  MeaModule6/1 -> Bus Creator/8
  MeaModule7/1 -> Bus Creator/9
  MeaModule8/1 -> Bus Creator/11
  MeaModule9/1 -> Bus Creator/1  "MCFL_ActualTorque"

== system VehCtrlMdel241025_2018b_amkspdlimit/Input/AMKMCU_Receive/FLAMKMCU/AMKMCU_state1/MCU_state ==
  ID : Inport
  Msg : Inport  Port=2
  Enable : EnablePort
  CAN Unpack : canmsglib/CAN Unpack  CANdbFile=d:\Users\YJR\Desktop\低压组\amk电机\DRe20_dbc_v1.16\DRe20_dbc_v1.16_CAN2.dbc  MsgList=(none)  MsgName=MCFL_ActualValue2  MsgIDType=Standard (11-bit identifier)  MsgIdentifier=642  MsgLength=8  SignalInfo={'MCFL_DiagnosticNum','0','32','LE','unsigned','Standard','0','1','0','-Inf','Inf';'MCFL_ErrorInfo','32','32','LE','unsigned','Standard','0','1','0','-Inf','Inf'}  IDPort=off  TimestampPort=off  ErrorPort=off  RemotePort=off  LengthPort=off  StatusPort=off  ApplyMinMax=off
      settings: SourceProductName=Simulink Real-Time  SourceProductBaseCode=XP  DataFormat=CANdb specified signals
  CANUnPackMessage4 : ec5744lib/RapidECU_U3/04CANCommunication/CANUnPackMessage  datalength=8  canmessagetype=Standard(11-bit ID)  sampletime=-1
      settings: SourceProductName=ECUCoder for MPC5744
  MeaModule1 : ec5744lib/RapidECU_U3/07Calibration/MeaModule  signal=MCFL_ErrorInfo
      settings: SourceProductName=ECUCoder for MPC5744
  MCFL_DiagnosticNum : Outport  VectorParamsAs1DForOutWhenUnconnected=off
  MCFL_ErrorInfo : Outport  Port=2  VectorParamsAs1DForOutWhenUnconnected=off
  wires:
  CANUnPackMessage4/1 -> CAN Unpack/1
  ID/1 -> CANUnPackMessage4/1
  Msg/1 -> CANUnPackMessage4/2
  CAN Unpack/1 -> MCFL_DiagnosticNum/1  "MCFL_DiagnosticNum"
  CAN Unpack/2 -> MeaModule1/1  "MCFL_ErrorInfo"
  MeaModule1/1 -> MCFL_ErrorInfo/1

== system VehCtrlMdel241025_2018b_amkspdlimit/Input/AMKMCU_Receive/FLAMKMCU/AMKMCU_state2/MCU_state ==
  ID : Inport
  Msg : Inport  Port=2
  Enable : EnablePort
  CAN Unpack : canmsglib/CAN Unpack  CANdbFile=d:\Users\YJR\Desktop\低压组\amk电机\DRe20_dbc_v1.16\DRe20_dbc_v1.16_CAN2.dbc  MsgList=(none)  MsgName=MCFL_ActualValue3  MsgIDType=Standard (11-bit identifier)  MsgIdentifier=644  MsgLength=6  SignalInfo={'MCFL_TempIGBT','32','16','LE','unsigned','Standard','0','0.1','0','-Inf','Inf';'MCFL_TempInverter','16','16','LE','unsigned','Standard','0','0.1','0','-Inf','Inf';'MCFL_TempMotor','0','16','LE','unsigned','Standard','0','0.1','0','-Inf','Inf'}  IDPort=off  TimestampPort=off  ErrorPort=off  RemotePort=off  LengthPort=off  StatusPort=off  ApplyMinMax=off
      settings: SourceProductName=Simulink Real-Time  SourceProductBaseCode=XP  DataFormat=CANdb specified signals
  CANUnPackMessage4 : ec5744lib/RapidECU_U3/04CANCommunication/CANUnPackMessage  datalength=6  canmessagetype=Standard(11-bit ID)  sampletime=-1
      settings: SourceProductName=ECUCoder for MPC5744
  MeaModule1 : ec5744lib/RapidECU_U3/07Calibration/MeaModule  signal=MCFL_TempIGBT
      settings: SourceProductName=ECUCoder for MPC5744
  MeaModule2 : ec5744lib/RapidECU_U3/07Calibration/MeaModule  signal=MCFL_TempInverter
      settings: SourceProductName=ECUCoder for MPC5744
  MeaModule3 : ec5744lib/RapidECU_U3/07Calibration/MeaModule  signal=MCFL_TempMotor
      settings: SourceProductName=ECUCoder for MPC5744
  MCFL_TempIGBT : Outport  VectorParamsAs1DForOutWhenUnconnected=off
  MCFL_TempInverter : Outport  Port=2  VectorParamsAs1DForOutWhenUnconnected=off
  MCFL_TempMotor : Outport  Port=3  VectorParamsAs1DForOutWhenUnconnected=off
  wires:
  Msg/1 -> CANUnPackMessage4/2
  ID/1 -> CANUnPackMessage4/1
  CANUnPackMessage4/1 -> CAN Unpack/1
  CAN Unpack/1 -> MeaModule1/1  "MCFL_TempIGBT"
  CAN Unpack/2 -> MeaModule2/1  "MCFL_TempInverter"
  CAN Unpack/3 -> MeaModule3/1  "MCFL_TempMotor"
  MeaModule1/1 -> MCFL_TempIGBT/1
  MeaModule2/1 -> MCFL_TempInverter/1
  MeaModule3/1 -> MCFL_TempMotor/1

== system VehCtrlMdel241025_2018b_amkspdlimit/Input/AMKMCU_Receive/FRAMKMCU/AMKMCU_state/MCU_state ==
  ID : Inport
  Msg : Inport  Port=2
  Enable : EnablePort
  CAN Unpack : canmsglib/CAN Unpack  CANdbFile=d:\Users\YJR\Desktop\低压组\amk电机\DRe20_dbc_v1.16\DRe20_dbc_v1.16_CAN2.dbc  MsgList=(none)  MsgName=MCFR_ActualValue1  MsgIDType=Standard (11-bit identifier)  MsgIdentifier=641  MsgLength=8  SignalInfo={'MCFR_ActualTorque','32','16','LE','signed','Standard','0','0.0098','0','-Inf','Inf';'MCFR_ActualVelocity','48','16','LE','signed','Standard','0','1','0','-Inf','Inf';'MCFR_DCVoltage','16','16','LE','unsigned','Standard','0','1','0','-Inf','Inf';'MCFR_bDCOn','12','1','LE','unsigned','Standard','0','1','0','0','1';'MCFR_bDerating','15','1','LE','unsigned','Standard','0','1','0','0','1';'MCFR_bError','9','1','LE','unsigned','Standard','0','1','0','0','1';'MCFR_bInverterOn','14','1','LE','unsigned','Standard','0','1','0','0','1';'MCFR_bQuitDCOn','11','1','LE','unsigned','Standard','0','1','0','0','1';'MCFR_bQuitInverterOn','13','1','LE','unsigned','Standard','0','1','0','0','1';'MCFR_bReserve','0','8','LE','unsigned','Standard','0','1','0','0','255';'MCFR_bSystemReady','8','1','LE','unsigned','Standard','0','1','0','0','1';'MCFR_bWarn','10','1','LE','unsigned','Standard','0','1','0','0','1'}  IDPort=off  TimestampPort=off  ErrorPort=off  RemotePort=off  LengthPort=off  StatusPort=off  ApplyMinMax=off
      settings: SourceProductName=Simulink Real-Time  SourceProductBaseCode=XP  DataFormat=CANdb specified signals
  CANUnPackMessage4 : ec5744lib/RapidECU_U3/04CANCommunication/CANUnPackMessage  datalength=8  canmessagetype=Standard(11-bit ID)  sampletime=-1
      settings: SourceProductName=ECUCoder for MPC5744
  MeaModule1 : ec5744lib/RapidECU_U3/07Calibration/MeaModule  signal=MCFR_ActualVelocity
      settings: SourceProductName=ECUCoder for MPC5744
  MeaModule2 : ec5744lib/RapidECU_U3/07Calibration/MeaModule  signal=MCFR_DCVoltage
      settings: SourceProductName=ECUCoder for MPC5744
  MeaModule3 : ec5744lib/RapidECU_U3/07Calibration/MeaModule  signal=MCFR_bDCOn
      settings: SourceProductName=ECUCoder for MPC5744
  MeaModule4 : ec5744lib/RapidECU_U3/07Calibration/MeaModule  signal=MCFR_bError
      settings: SourceProductName=ECUCoder for MPC5744
  MeaModule5 : ec5744lib/RapidECU_U3/07Calibration/MeaModule  signal=MCFR_bInverterOn
      settings: SourceProductName=ECUCoder for MPC5744
  MeaModule6 : ec5744lib/RapidECU_U3/07Calibration/MeaModule  signal=MCFR_bQuitInverterOn
      settings: SourceProductName=ECUCoder for MPC5744
  MeaModule7 : ec5744lib/RapidECU_U3/07Calibration/MeaModule  signal=MCFR_bSystemReady
      settings: SourceProductName=ECUCoder for MPC5744
  MeaModule8 : ec5744lib/RapidECU_U3/07Calibration/MeaModule  signal=MCFR_ActualTorque
      settings: SourceProductName=ECUCoder for MPC5744
  MCFR_ActualTorque : Outport  VectorParamsAs1DForOutWhenUnconnected=off
  MCFR_ActualVelocity : Outport  Port=2  VectorParamsAs1DForOutWhenUnconnected=off
  MCFR_DCVoltage : Outport  Port=3  VectorParamsAs1DForOutWhenUnconnected=off
  MCFR_bDCOn : Outport  Port=4  VectorParamsAs1DForOutWhenUnconnected=off
  MCFR_bDerating : Outport  Port=5  VectorParamsAs1DForOutWhenUnconnected=off
  MCFR_bError : Outport  Port=6  VectorParamsAs1DForOutWhenUnconnected=off
  MCFR_bInverterOn : Outport  Port=7  VectorParamsAs1DForOutWhenUnconnected=off
  MCFR_bQuitDCOn : Outport  Port=8  VectorParamsAs1DForOutWhenUnconnected=off
  MCFR_bQuitInverterOn : Outport  Port=9  VectorParamsAs1DForOutWhenUnconnected=off
  MCFR_bReserve : Outport  Port=10  VectorParamsAs1DForOutWhenUnconnected=off
  MCFR_bSystemReady : Outport  Port=11  VectorParamsAs1DForOutWhenUnconnected=off
  MCFR_bWarn : Outport  Port=12  VectorParamsAs1DForOutWhenUnconnected=off
  wires:
  CANUnPackMessage4/1 -> CAN Unpack/1
  ID/1 -> CANUnPackMessage4/1
  Msg/1 -> CANUnPackMessage4/2
  CAN Unpack/1 -> MeaModule8/1  "MCFR_ActualTorque"
  CAN Unpack/2 -> MeaModule1/1  "MCFR_ActualVelocity"
  CAN Unpack/4 -> MeaModule3/1  "MCFR_bDCOn"
  CAN Unpack/3 -> MeaModule2/1  "MCFR_DCVoltage"
  CAN Unpack/7 -> MeaModule5/1  "MCFR_bInverterOn"
  CAN Unpack/5 -> MCFR_bDerating/1  "MCFR_bDerating"
  CAN Unpack/6 -> MeaModule4/1  "MCFR_bError"
  CAN Unpack/8 -> MCFR_bQuitDCOn/1  "MCFR_bQuitDCOn"
  CAN Unpack/9 -> MeaModule6/1  "MCFR_bQuitInverterOn"
  CAN Unpack/10 -> MCFR_bReserve/1  "MCFR_bReserve"
  CAN Unpack/11 -> MeaModule7/1  "MCFR_bSystemReady"
  CAN Unpack/12 -> MCFR_bWarn/1  "MCFR_bWarn"
  MeaModule1/1 -> MCFR_ActualVelocity/1
  MeaModule2/1 -> MCFR_DCVoltage/1
  MeaModule3/1 -> MCFR_bDCOn/1
  MeaModule4/1 -> MCFR_bError/1
  MeaModule5/1 -> MCFR_bInverterOn/1
  MeaModule6/1 -> MCFR_bQuitInverterOn/1
  MeaModule7/1 -> MCFR_bSystemReady/1
  MeaModule8/1 -> MCFR_ActualTorque/1  "MCFR_ActualTorque"

== system VehCtrlMdel241025_2018b_amkspdlimit/Input/AMKMCU_Receive/FRAMKMCU/AMKMCU_state1/MCU_state ==
  ID : Inport
  Msg : Inport  Port=2
  Enable : EnablePort
  CAN Unpack : canmsglib/CAN Unpack  CANdbFile=d:\Users\YJR\Desktop\低压组\amk电机\DRe20_dbc_v1.16\DRe20_dbc_v1.16_CAN2.dbc  MsgList=(none)  MsgName=MCFR_ActualValue2  MsgIDType=Standard (11-bit identifier)  MsgIdentifier=643  MsgLength=8  SignalInfo={'MCFR_DiagnosticNum','0','32','LE','unsigned','Standard','0','1','0','-Inf','Inf';'MCFR_ErrorInfo','32','32','LE','unsigned','Standard','0','1','0','-Inf','Inf'}  IDPort=off  TimestampPort=off  ErrorPort=off  RemotePort=off  LengthPort=off  StatusPort=off  ApplyMinMax=off
      settings: SourceProductName=Simulink Real-Time  SourceProductBaseCode=XP  DataFormat=CANdb specified signals
  CANUnPackMessage4 : ec5744lib/RapidECU_U3/04CANCommunication/CANUnPackMessage  datalength=8  canmessagetype=Standard(11-bit ID)  sampletime=-1
      settings: SourceProductName=ECUCoder for MPC5744
  MeaModule1 : ec5744lib/RapidECU_U3/07Calibration/MeaModule  signal=MCFR_ErrorInfo
      settings: SourceProductName=ECUCoder for MPC5744
  MCFR_DiagnosticNum : Outport  VectorParamsAs1DForOutWhenUnconnected=off
  MCFR_ErrorInfo : Outport  Port=2  VectorParamsAs1DForOutWhenUnconnected=off
  wires:
  Msg/1 -> CANUnPackMessage4/2
  ID/1 -> CANUnPackMessage4/1
  CANUnPackMessage4/1 -> CAN Unpack/1
  CAN Unpack/1 -> MCFR_DiagnosticNum/1  "MCFR_DiagnosticNum"
  CAN Unpack/2 -> MeaModule1/1  "MCFR_ErrorInfo"
  MeaModule1/1 -> MCFR_ErrorInfo/1

== system VehCtrlMdel241025_2018b_amkspdlimit/Input/AMKMCU_Receive/FRAMKMCU/AMKMCU_state2/MCU_state ==
  ID : Inport
  Msg : Inport  Port=2
  Enable : EnablePort
  CAN Unpack : canmsglib/CAN Unpack  CANdbFile=d:\Users\YJR\Desktop\低压组\amk电机\DRe20_dbc_v1.16\DRe20_dbc_v1.16_CAN2.dbc  MsgList=(none)  MsgName=MCFR_ActualValue3  MsgIDType=Standard (11-bit identifier)  MsgIdentifier=645  MsgLength=6  SignalInfo={'MCFR_TempIGBT','32','16','LE','unsigned','Standard','0','0.1','0','-Inf','Inf';'MCFR_TempInverter','16','16','LE','unsigned','Standard','0','0.1','0','-Inf','Inf';'MCFR_TempMotor','0','16','LE','unsigned','Standard','0','0.1','0','-Inf','Inf'}  IDPort=off  TimestampPort=off  ErrorPort=off  RemotePort=off  LengthPort=off  StatusPort=off  ApplyMinMax=off
      settings: SourceProductName=Simulink Real-Time  SourceProductBaseCode=XP  DataFormat=CANdb specified signals
  CANUnPackMessage4 : ec5744lib/RapidECU_U3/04CANCommunication/CANUnPackMessage  datalength=6  canmessagetype=Standard(11-bit ID)  sampletime=-1
      settings: SourceProductName=ECUCoder for MPC5744
  MeaModule1 : ec5744lib/RapidECU_U3/07Calibration/MeaModule  signal=MCFR_TempIGBT
      settings: SourceProductName=ECUCoder for MPC5744
  MeaModule2 : ec5744lib/RapidECU_U3/07Calibration/MeaModule  signal=MCFR_TempInverter
      settings: SourceProductName=ECUCoder for MPC5744
  MeaModule3 : ec5744lib/RapidECU_U3/07Calibration/MeaModule  signal=MCFR_TempMotor
      settings: SourceProductName=ECUCoder for MPC5744
  MCFR_TempIGBT : Outport  VectorParamsAs1DForOutWhenUnconnected=off
  MCFR_TempInverter : Outport  Port=2  VectorParamsAs1DForOutWhenUnconnected=off
  MCFR_TempMotor : Outport  Port=3  VectorParamsAs1DForOutWhenUnconnected=off
  wires:
  CANUnPackMessage4/1 -> CAN Unpack/1
  ID/1 -> CANUnPackMessage4/1
  Msg/1 -> CANUnPackMessage4/2
  CAN Unpack/1 -> MeaModule1/1  "MCFR_TempIGBT"
  CAN Unpack/2 -> MeaModule2/1  "MCFR_TempInverter"
  CAN Unpack/3 -> MeaModule3/1  "MCFR_TempMotor"
  MeaModule1/1 -> MCFR_TempIGBT/1
  MeaModule2/1 -> MCFR_TempInverter/1
  MeaModule3/1 -> MCFR_TempMotor/1

== system VehCtrlMdel241025_2018b_amkspdlimit/Input_Processing/Subsystem/WhlSlpageJudgment/加速度差判断/Filter ==
  In : Inport
  Add : Sum
  Constant : Constant  Value=single(-100)
  Constant1 : Constant  Value=single(100)
  Constant2 : Constant  Value=single(100)
  Constant3 : Constant  Value=single(-100)
  Gain : Gain  Gain=0.3
  Gain1 : Gain  Gain=0.7
  Rate Limiter Dynamic : simulink/Discontinuities/Rate Limiter Dynamic
      settings: SourceProductName=Simulink
  Saturation Dynamic : simulink/Discontinuities/Saturation Dynamic  OutMin=[]  OutMax=[]  OutDataTypeStr=Inherit: Same as second input  OutDataType=fixdt(1, 16)  OutScaling=2^-10  DoSatur=off
  Unit Delay : UnitDelay  SampleTime=-1  HasFrameUpgradeWarning=on
  Out : Outport
  wires:
  In/1 -> Saturation Dynamic/2
  Saturation Dynamic/1 -> Rate Limiter Dynamic/2
  Constant1/1 -> Saturation Dynamic/1
  Constant/1 -> Saturation Dynamic/3
  Constant2/1 -> Rate Limiter Dynamic/1
  Constant3/1 -> Rate Limiter Dynamic/3
  Unit Delay/1 -> Gain/1
  Gain/1 -> Add/1
  Add/1 -> Out/1
  Gain1/1 -> Add/2
  Rate Limiter Dynamic/1 -> Gain1/1, Unit Delay/1

== system VehCtrlMdel241025_2018b_amkspdlimit/Input_Processing/Subsystem/WhlSlpageJudgment/加速度差判断/Filter1 ==
  In : Inport
  Add : Sum
  Constant : Constant  Value=single(-100)
  Constant1 : Constant  Value=single(100)
  Constant2 : Constant  Value=single(100)
  Constant3 : Constant  Value=single(-100)
  Gain : Gain  Gain=0.3
  Gain1 : Gain  Gain=0.7
  Rate Limiter Dynamic : simulink/Discontinuities/Rate Limiter Dynamic
      settings: SourceProductName=Simulink
  Saturation Dynamic : simulink/Discontinuities/Saturation Dynamic  OutMin=[]  OutMax=[]  OutDataTypeStr=Inherit: Same as second input  OutDataType=fixdt(1, 16)  OutScaling=2^-10  DoSatur=off
  Unit Delay : UnitDelay  SampleTime=-1  HasFrameUpgradeWarning=on
  Out : Outport
  wires:
  Rate Limiter Dynamic/1 -> Unit Delay/1, Gain1/1
  Gain1/1 -> Add/2
  Add/1 -> Out/1
  Gain/1 -> Add/1
  Unit Delay/1 -> Gain/1
  Constant3/1 -> Rate Limiter Dynamic/3
  Constant2/1 -> Rate Limiter Dynamic/1
  Constant/1 -> Saturation Dynamic/3
  Constant1/1 -> Saturation Dynamic/1
  Saturation Dynamic/1 -> Rate Limiter Dynamic/2
  In/1 -> Saturation Dynamic/2

== system VehCtrlMdel241025_2018b_amkspdlimit/Input_Processing/Subsystem/WhlSlpageJudgment/加速度差判断/Filter2 ==
  In : Inport
  Add : Sum
  Constant : Constant  Value=single(-100)
  Constant1 : Constant  Value=single(100)
  Constant2 : Constant  Value=single(100)
  Constant3 : Constant  Value=single(-100)
  Gain : Gain  Gain=0.3
  Gain1 : Gain  Gain=0.7
  Rate Limiter Dynamic : simulink/Discontinuities/Rate Limiter Dynamic
      settings: SourceProductName=Simulink
  Saturation Dynamic : simulink/Discontinuities/Saturation Dynamic  OutMin=[]  OutMax=[]  OutDataTypeStr=Inherit: Same as second input  OutDataType=fixdt(1, 16)  OutScaling=2^-10  DoSatur=off
  Unit Delay : UnitDelay  SampleTime=-1  HasFrameUpgradeWarning=on
  Out : Outport
  wires:
  In/1 -> Saturation Dynamic/2
  Saturation Dynamic/1 -> Rate Limiter Dynamic/2
  Constant1/1 -> Saturation Dynamic/1
  Constant/1 -> Saturation Dynamic/3
  Constant2/1 -> Rate Limiter Dynamic/1
  Constant3/1 -> Rate Limiter Dynamic/3
  Unit Delay/1 -> Gain/1
  Gain/1 -> Add/1
  Add/1 -> Out/1
  Gain1/1 -> Add/2
  Rate Limiter Dynamic/1 -> Gain1/1, Unit Delay/1

== system VehCtrlMdel241025_2018b_amkspdlimit/Input_Processing/Subsystem/WhlSlpageJudgment/加速度差判断/Filter3 ==
  In : Inport
  Add : Sum
  Constant : Constant  Value=single(-100)
  Constant1 : Constant  Value=single(100)
  Constant2 : Constant  Value=single(100)
  Constant3 : Constant  Value=single(-100)
  Gain : Gain  Gain=0.3
  Gain1 : Gain  Gain=0.7
  Rate Limiter Dynamic : simulink/Discontinuities/Rate Limiter Dynamic
      settings: SourceProductName=Simulink
  Saturation Dynamic : simulink/Discontinuities/Saturation Dynamic  OutMin=[]  OutMax=[]  OutDataTypeStr=Inherit: Same as second input  OutDataType=fixdt(1, 16)  OutScaling=2^-10  DoSatur=off
  Unit Delay : UnitDelay  SampleTime=-1  HasFrameUpgradeWarning=on
  Out : Outport
  wires:
  Rate Limiter Dynamic/1 -> Unit Delay/1, Gain1/1
  Gain1/1 -> Add/2
  Add/1 -> Out/1
  Gain/1 -> Add/1
  Unit Delay/1 -> Gain/1
  Constant3/1 -> Rate Limiter Dynamic/3
  Constant2/1 -> Rate Limiter Dynamic/1
  Constant/1 -> Saturation Dynamic/3
  Constant1/1 -> Saturation Dynamic/1
  Saturation Dynamic/1 -> Rate Limiter Dynamic/2
  In/1 -> Saturation Dynamic/2

== system VehCtrlMdel241025_2018b_amkspdlimit/Input_Processing/Subsystem/WhlSlpageJudgment/加速度差的微分的判断/Filter ==
  In : Inport
  Add : Sum
  Constant : Constant  Value=single(-100)
  Constant1 : Constant  Value=single(100)
  Constant2 : Constant  Value=single(20)
  Constant3 : Constant  Value=single(-20)
  Gain : Gain  Gain=0.5
  Gain1 : Gain  Gain=0.5
  Rate Limiter Dynamic : simulink/Discontinuities/Rate Limiter Dynamic
      settings: SourceProductName=Simulink
  Saturation Dynamic : simulink/Discontinuities/Saturation Dynamic  OutMin=[]  OutMax=[]  OutDataTypeStr=Inherit: Same as second input  OutDataType=fixdt(1, 16)  OutScaling=2^-10  DoSatur=off
  Unit Delay : UnitDelay  SampleTime=-1  HasFrameUpgradeWarning=on
  Out : Outport
  wires:
  In/1 -> Saturation Dynamic/2
  Saturation Dynamic/1 -> Rate Limiter Dynamic/2
  Constant1/1 -> Saturation Dynamic/1
  Constant/1 -> Saturation Dynamic/3
  Constant2/1 -> Rate Limiter Dynamic/1
  Constant3/1 -> Rate Limiter Dynamic/3
  Unit Delay/1 -> Gain/1
  Gain/1 -> Add/1
  Add/1 -> Out/1
  Gain1/1 -> Add/2
  Rate Limiter Dynamic/1 -> Gain1/1, Unit Delay/1

== system VehCtrlMdel241025_2018b_amkspdlimit/Input_Processing/Subsystem/WhlSlpageJudgment/加速度差的微分的判断/Filter1 ==
  In : Inport
  Add : Sum
  Constant : Constant  Value=single(-100)
  Constant1 : Constant  Value=single(100)
  Constant2 : Constant  Value=single(20)
  Constant3 : Constant  Value=single(-20)
  Gain : Gain  Gain=0.5
  Gain1 : Gain  Gain=0.5
  Rate Limiter Dynamic : simulink/Discontinuities/Rate Limiter Dynamic
      settings: SourceProductName=Simulink
  Saturation Dynamic : simulink/Discontinuities/Saturation Dynamic  OutMin=[]  OutMax=[]  OutDataTypeStr=Inherit: Same as second input  OutDataType=fixdt(1, 16)  OutScaling=2^-10  DoSatur=off
  Unit Delay : UnitDelay  SampleTime=-1  HasFrameUpgradeWarning=on
  Out : Outport
  wires:
  Rate Limiter Dynamic/1 -> Unit Delay/1, Gain1/1
  Gain1/1 -> Add/2
  Add/1 -> Out/1
  Gain/1 -> Add/1
  Unit Delay/1 -> Gain/1
  Constant3/1 -> Rate Limiter Dynamic/3
  Constant2/1 -> Rate Limiter Dynamic/1
  Constant/1 -> Saturation Dynamic/3
  Constant1/1 -> Saturation Dynamic/1
  Saturation Dynamic/1 -> Rate Limiter Dynamic/2
  In/1 -> Saturation Dynamic/2
